simulink model "Commande_3_Changement_de_base_et_diffeomorphisme_"  (R2015a)
settings: Solver=ode45  StartTime=0.0  StopTime=15  MaxStep=0.001  RelTol=1e-3
values from neighbouring files (symbols this model uses):
  Ks = K(:,4)    [A_2_Changement_de_base_Diphiomorphisme.m]
  Kw = K( : , 1:3 )    [A_2_Changement_de_base_Diphiomorphisme.m]
undefined symbols (not defined in the file or in its folder): sfun3d
settings Model: Creator=user  LastModifiedBy=user

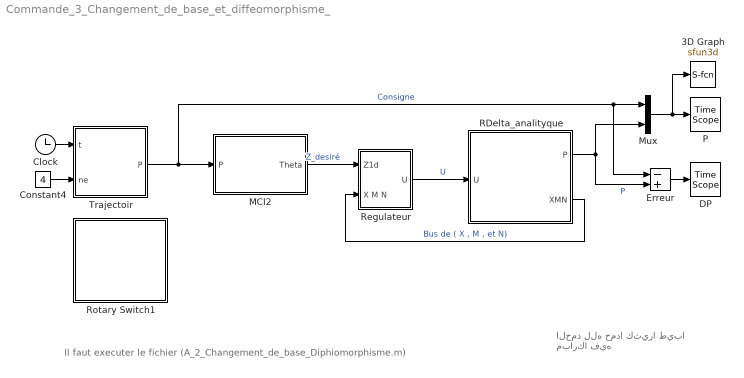
== system Commande_3_Changement_de_base_et_diffeomorphisme_ ==
  note: Il faut executer le fichier (A_2_Changement_de_base_Diphiomorphisme.m)
  note: الحمد لله حمدا كثيرا طيبا مباركا فيه
  3D Graph : S-Function  LoadFcn=sfun3d([],[],[],'LoadBlock')  StartFcn=sfun3d([],[],[],'Start')  StopFcn=sfun3d([],[],[],'Stop')  FunctionName=sfun3d  Parameters=ax,T,np,cp,gd,ls,mk  mask(3D Graph){np=2, ax=[-1 1 -1 1 -2 0]*0.3, cp=[3 2 1], gd=on, ls=-, mk=none, T=0.0001}
      mask prompts: np "Number of point (lines)"; ax "[xmin xmax  ymin ymax zmin zmax]"; cp "Camera position (use [0 0 1] for 2D XY view)"; gd "Grid (on|off)"; ls "LineStyle"; mk "Marker"; T "Sampling Time"
      mask help:
      | This block plots the position of several points in the XYZ space. The input contains the coordinates of all the points (x1,y1,z1,x2,y2,z2,...).
      | The number of points (lines), the XYZ ranges, camera position, grid, linestyle, marker and sampling time, can be set as mask parameters.
      settings: CopyFcn=sfun3d([],[],[],'CopyBlock')  DeleteFcn=sfun3d([],[],[],'DeleteBlock')  NameChangeFcn=sfun3d([],[],[],'NameChange')
      mask Help:
      | This block plots the position of several points in the XYZ space. The input contains the coordinates of all the points (x1,y1,z1,x2,y2,z2,...).
      | The number of points (lines), the XYZ ranges, camera position, grid, linestyle, marker and sampling time, can be set as mask parameters.
      mask TypeOptions ls: - | -- | : | -. | none
      mask TypeOptions mk: none | . | + | o | * | x | square | diamond | v | ^ | > | < | pentagram | hexagram
      mask Display: plot([.05 .95 .95 .05 .05],[.45 .45 .95 .95 .45], 0.5+cos(0:0.1:2*pi)*0.3,0.7+sin(0:0.1:2*pi)*0.2)
  Clock : Clock
  Constant4 : Constant  Value=4
  DP : TimeScope  DefaultConfigurationName=spbscopes.TimeScopeBlockCfg
  Erreur : Sum  Inputs=-+
  MCI2 : MATLAB Function  TreatAsAtomicUnit=on
  Mux : Mux  Inputs=2
  P : TimeScope  DefaultConfigurationName=spbscopes.TimeScopeBlockCfg
  RDelta_analityque : Subsystem
      mask Display:
      | image(imread('DeltaImage2.PNG'))
      | 
      | port_label('input',1,'U')
      | 
      | port_label('output',1,'P')
      | 
      | port_label('output',2,'XMN')
  Regulateur : Subsystem
  Rotary Switch1 : Subsystem  DialogController=hmiCreateDDGDialog  IsWebBlock=on  mask(MathWorksWebBlock){webBlockId=e030fcf6-dd97-4258-a719-13022b0e8ecf, webBlockType=discreteknob, ShowInLibBrowser=on, ShowInitialText=on, HMISrcModelName=Commande_3_Changement_de_base_et_diffeomorphisme_}
      mask prompts: webBlockId "WebBlock Id"; webBlockType "WebBlock Type"; HMISrcModelName "Source Model"
      mask Help: helpview([docroot '/mapfiles/simulink.map'], 'hmi_rotary_switch')
      mask Display:
      | model = bdroot(gcb);
      | if strcmp(get_param(model,'BlockDiagramType'), 'library')
      |     image([(matlabroot) '/toolbox/simulink/hmi/icons/DiscreteKnob.png']);
      | end
  Trajectoir : MATLAB Function  TreatAsAtomicUnit=on
  wires:
  RDelta_analityque/1(P) -> Erreur/2, Mux/2  "P"
  Mux/1 -> P/1, 3D Graph/1
  RDelta_analityque/2(XMN) -> Regulateur/2(X M N)  "Bus de ( X , M , et N)"
  Regulateur/1(U) -> RDelta_analityque/1(U)  "U"
  Trajectoir/1(P) -> MCI2/1(P), Mux/1, Erreur/1  "Consigne"
  Clock/1 -> Trajectoir/1(t)
  Constant4/1 -> Trajectoir/2(ne)
  MCI2/1(Theta) -> Regulateur/1(Z1d)  "Z_desiré"
  Erreur/1 -> DP/1

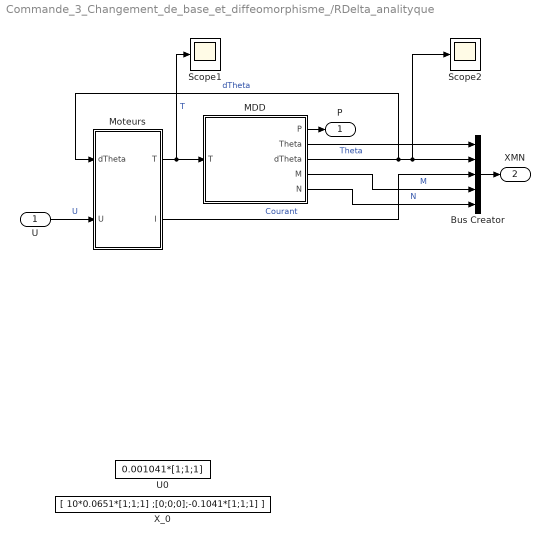
== system Commande_3_Changement_de_base_et_diffeomorphisme_/RDelta_analityque ==
  U : Inport
  Bus Creator : BusCreator  Inputs=5
  MDD : Subsystem
      mask Display:
      | image(imread('DeltaImage2.PNG'))
      | port_label('input',1,'T')
      | port_label('output',1,'P')
      | port_label('output',2,'Theta')
      | port_label('output',3,'dTheta')
      | port_label('output',4,'M')
      | port_label('output',5,'N')
  Moteurs : Subsystem
      mask Display:
      | image('image_motor.jpg')
      | port_label('output',1,'T')
      | port_label('output',2,'I')
      | port_label('input',1,'U')
      | port_label('input',2,'dTheta')
  Scope1 : Scope
      settings: YMin=-0.2  YMax=0.175  SaveName=ScopeData3
  Scope2 : Scope
      settings: YMin=0.774525  YMax=0.774531  SaveName=ScopeData7
  U0 : Constant  Value=0.001041*[1;1;1]
  X_0 : Constant  Value=[ 10*0.0651*[1;1;1] ;[0;0;0];-0.1041*[1;1;1] ]
  P : Outport
  XMN : Outport  Port=2
  wires:
  Moteurs/2(I) -> Bus Creator/3  "Courant"
  U/1 -> Moteurs/2(U)  "U"
  MDD/2(Theta) -> Bus Creator/1  "Theta"
  MDD/3(dTheta) -> Moteurs/1(dTheta), Bus Creator/2, Scope2/1  "dTheta"
  Moteurs/1(T) -> Scope1/1, MDD/1(T)  "T"
  MDD/1(P) -> P/1
  MDD/4(M) -> Bus Creator/4  "M"
  MDD/5(N) -> Bus Creator/5  "N"
  Bus Creator/1 -> XMN/1

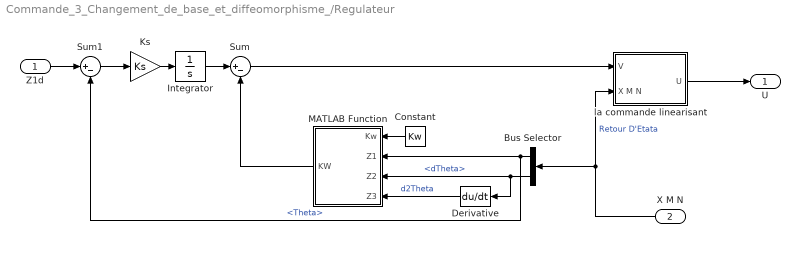
== system Commande_3_Changement_de_base_et_diffeomorphisme_/Regulateur ==
  Z1d : Inport
  X M N : Inport  Port=2
  Bus Selector : BusSelector  OutputSignals=Theta,dTheta
  Constant : Constant  Value=Kw
  Derivative : Derivative
  Integrator : Integrator
  Ks : Gain  Gain=Ks
  MATLAB Function : MATLAB Function  TreatAsAtomicUnit=on
  Sum : Sum  Inputs=|+-
  Sum1 : Sum  Inputs=|+-
  la commande linearisant : Subsystem
  U : Outport
  wires:
  la commande linearisant/1(U) -> U/1
  Derivative/1 -> MATLAB Function/4(Z3)  "d2Theta"
  Bus Selector/1 -> MATLAB Function/2(Z1), Sum1/2  "<Theta>"
  X M N/1 -> Bus Selector/1, la commande linearisant/2(X M N)  "Retour D'Etata"
  Bus Selector/2 -> MATLAB Function/3(Z2), Derivative/1  "<dTheta>"
  Ks/1 -> Integrator/1
  MATLAB Function/1(KW) -> Sum/2
  Sum/1 -> la commande linearisant/1(V)
  Integrator/1 -> Sum/1
  Z1d/1 -> Sum1/1
  Sum1/1 -> Ks/1
  Constant/1 -> MATLAB Function/1(Kw)

== system Commande_3_Changement_de_base_et_diffeomorphisme_/Rotary Switch1 ==

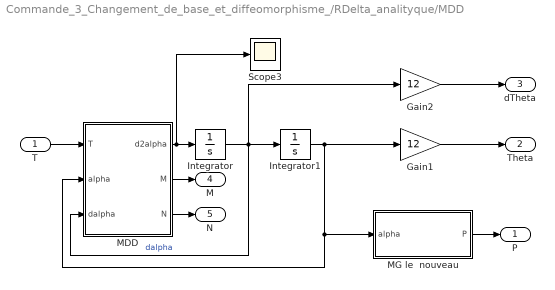
== system Commande_3_Changement_de_base_et_diffeomorphisme_/RDelta_analityque/MDD ==
  T : Inport
  Gain1 : Gain  Gain=12
  Gain2 : Gain  Gain=12
  Integrator : Integrator  InitialCondition=[0;0;0]
  Integrator1 : Integrator  InitialCondition=0.8*[1;1;1]/12
  MDD : Subsystem
  MG le  nouveau : MATLAB Function  TreatAsAtomicUnit=on
  Scope3 : Scope
      settings: TimeRange=2.077341948455237  YMin=0.00075  YMax=0.00275  SaveName=ScopeData2
  P : Outport
  Theta : Outport  Port=2
  dTheta : Outport  Port=3
  M : Outport  Port=4
  N : Outport  Port=5
  wires:
  MDD/1(d2alpha) -> Scope3/1, Integrator/1
  Integrator/1 -> Gain2/1, MDD/3(dalpha), Integrator1/1  "dalpha"
  Integrator1/1 -> MG le  nouveau/1(alpha), MDD/2(alpha), Gain1/1
  T/1 -> MDD/1(T)
  MG le  nouveau/1(P) -> P/1
  Gain1/1 -> Theta/1
  Gain2/1 -> dTheta/1
  MDD/2(M) -> M/1
  MDD/3(N) -> N/1

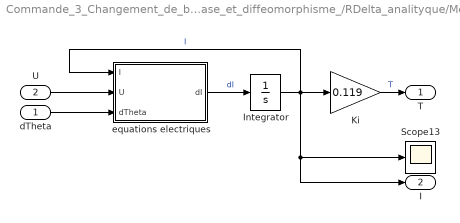
== system Commande_3_Changement_de_base_et_diffeomorphisme_/RDelta_analityque/Moteurs ==
  dTheta : Inport
  U : Inport  Port=2
  Integrator : Integrator  InitialCondition=0*[1;1;1]
  Ki : Gain  Gain=0.119
  Scope13 : Scope
      settings: TimeRange=0.507510643892459  YMin=-1000  YMax=1000  SaveName=ScopeData24
  equations electriques : MATLAB Function  TreatAsAtomicUnit=on
  T : Outport
  I : Outport  Port=2
  wires:
  U/1 -> equations electriques/2(U)
  Integrator/1 -> Scope13/1, I/1, Ki/1, equations electriques/1(I)  "I"
  equations electriques/1(dI) -> Integrator/1  "dI"
  dTheta/1 -> equations electriques/3(dTheta)
  Ki/1 -> T/1  "T"

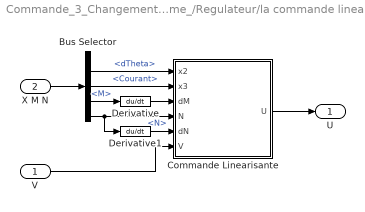
== system Commande_3_Changement_de_base_et_diffeomorphisme_/Regulateur/la commande linearisant ==
  V : Inport
  X M N : Inport  Port=2
  Bus Selector : BusSelector  OutputSignals=Theta,dTheta,Courant,M,N
  Commande Linearisante : MATLAB Function  TreatAsAtomicUnit=on
  Derivative : Derivative
  Derivative1 : Derivative
  U : Outport
  wires:
  X M N/1 -> Bus Selector/1
  Bus Selector/2 -> Commande Linearisante/1(x2)  "<dTheta>"
  Bus Selector/3 -> Commande Linearisante/2(x3)  "<Courant>"
  Derivative/1 -> Commande Linearisante/3(dM)
  Bus Selector/4 -> Derivative/1  "<M>"
  Derivative1/1 -> Commande Linearisante/5(dN)
  Bus Selector/5 -> Derivative1/1, Commande Linearisante/4(N)  "<N>"
  V/1 -> Commande Linearisante/6(V)
  Commande Linearisante/1(U) -> U/1

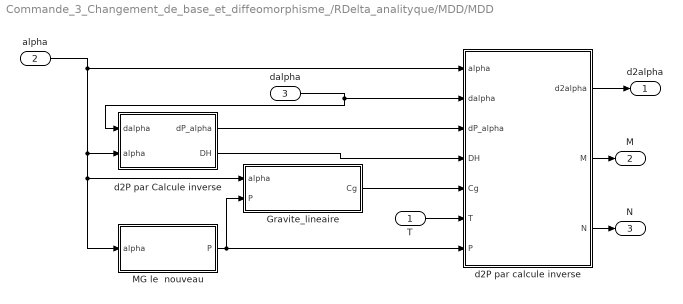
== system Commande_3_Changement_de_base_et_diffeomorphisme_/RDelta_analityque/MDD/MDD ==
  T : Inport
  alpha : Inport  Port=2
  dalpha : Inport  Port=3
  Gravite_lineaire : MATLAB Function  TreatAsAtomicUnit=on
  MG le  nouveau : MATLAB Function  TreatAsAtomicUnit=on
  "d2P par Calcule inverse " : Subsystem
  d2P par calcule inverse : MATLAB Function  TreatAsAtomicUnit=on
  d2alpha : Outport
  M : Outport  Port=2
  N : Outport  Port=3
  wires:
  d2P par calcule inverse/1(d2alpha) -> d2alpha/1
  "d2P par Calcule inverse "/1(dP_alpha) -> d2P par calcule inverse/3(dP_alpha)
  "d2P par Calcule inverse "/2(DH) -> d2P par calcule inverse/4(DH)
  MG le  nouveau/1(P) -> Gravite_lineaire/2(P), d2P par calcule inverse/7(P)
  dalpha/1 -> "d2P par Calcule inverse "/1(dalpha), d2P par calcule inverse/2(dalpha)
  alpha/1 -> MG le  nouveau/1(alpha), Gravite_lineaire/1(alpha), "d2P par Calcule inverse "/2(alpha), d2P par calcule inverse/1(alpha)
  Gravite_lineaire/1(Cg) -> d2P par calcule inverse/5(Cg)
  T/1 -> d2P par calcule inverse/6(T)
  d2P par calcule inverse/2(M) -> M/1
  d2P par calcule inverse/3(N) -> N/1

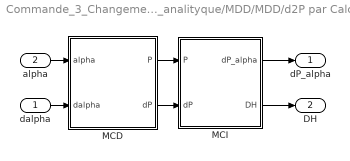
== system Commande_3_Changement_de_base_et_diffeomorphisme_/RDelta_analityque/MDD/MDD/d2P par Calcule inverse  ==
  dalpha : Inport
  alpha : Inport  Port=2
  MCD : MATLAB Function  TreatAsAtomicUnit=on
  MCI : MATLAB Function  TreatAsAtomicUnit=on
  dP_alpha : Outport
  DH : Outport  Port=2
  wires:
  MCD/2(dP) -> MCI/2(dP)
  MCD/1(P) -> MCI/1(P)
  alpha/1 -> MCD/1(alpha)
  dalpha/1 -> MCD/2(dalpha)
  MCI/1(dP_alpha) -> dP_alpha/1
  MCI/2(DH) -> DH/1

== matlab function Commande_3_Changement_de_base_et_diffeomorphisme_/RDelta_analityque/MDD/MDD/MG le  nouveau ==
  data: alpha input; P output
function P =MGD(alpha)


alpha1=alpha(1) ;alpha2=alpha(2) ; alpha3=alpha(3) ;

%les constantes
l1 = 0.19992; 
l2 = 0.334; 
r = 0.126; 
phi2 = 2*pi/3;
phi3 = 4*pi/3;

%% Les points :
C1=[r+l1*cos(alpha1) ; 0 ; -l1*sin(alpha1) ]; 
C2=[(r+l1*cos(alpha2))*cos(phi2) ; (r+l1*cos(alpha2))*sin(phi2) ; -l1*sin(alpha2) ]; 
C3=[(r+l1*cos(alpha3))*cos(phi3) ; (r+l1*cos(alpha3))*sin(phi3) ; -l1*sin(alpha3) ]; 

%% Les vecteurs du triangle C1C2C3 et ses distances
C1C2= C2-C1 ; C2C3 =C3-C2 ; C3C1= C1-C3 ;
a=sqrt(C1C2'*C1C2) ; b=sqrt(C2C3'*C2C3)  ; c=sqrt(C3C1'*C3C1)  ;
 p= a+b+c ; % Le perimetre de C1C2C3
 R = a*b*c/sqrt(p*(p-2*a)*(p-2*b)*(p-2*c)) ;

 %% Calcule du point L 
 % Les vecteurs u et n:
 v1=C1C2/a ;
 n=cross(C3C1,C1C2)*2*R/(a*b*c) ;
 TL = sqrt(R^2-a^2/4) ;
 OL=(C1+C2)/2+TL*sign(-a*a+c*c+b*b)*cross(n,v1);
 %% Calcule du point E :
P=OL-sqrt(l2^2-R^2)*n ;

== matlab function Commande_3_Changement_de_base_et_diffeomorphisme_/MCI2 ==
  data: P input; Theta output
    function Theta = fcn(P)

    l1 = 0.19992; 
    l2 = 0.334; 
    r = 0.126; 
    phi2 = 2*pi/3;
    phi3 = 4*pi/3;

    %% Expression de P dans Ri
    % l'expression P1 dP1 et d2P1 ne se changent pas
    A2=[cos(phi2) sin(phi2) 0
        -sin(phi2) cos(phi2) 0
        0            0      1 ]; 
    A3=[cos(phi3) sin(phi3) 0
        -sin(phi3) cos(phi3) 0
        0            0      1 ];
     P2=A2*P; 
     P3=A3*P ; 
        
    x1=P(1); y1=P(2) ; z1=P(3) ; 
    x2=P2(1); y2=P2(2) ; z2=P2(3) ;
    x3=P3(1); y3=P3(2) ; z3=P3(3) ;
   
    % L'expression de dP dans Ri :
      

    %% Parametres du Triangle AiCiBi :
    % Triangle 1 :
    AB1=sqrt(z1^2+(x1-r)^2);
    e1=sqrt(l2^2-y1^2); 
    AB2=sqrt(z2^2+(x2-r)^2);
    e2=sqrt(l2^2-y2^2);
    AB3=sqrt(z3^2+(x3-r)^2);
    e3=sqrt(l2^2-y3^2);

    %% calcul de alpha1
    beta1=atan2(-z1,x1-r);
    delta1=acos((AB1^2 + l1^2 - e1^2)/(2*l1*AB1));
    alpha1=beta1-delta1; 


    %% calcul de alpha2
    beta2=atan2(-z2,x2-r);
    delta2=acos((AB2^2 + l1^2 - e2^2)/(2*l1*AB2));
    alpha2=beta2-delta2; 


    %% calcul de alpha3
    beta3=atan2(-z3,x3-r);
    delta3=acos((AB3^2 + l1^2 - e3^2)/(2*l1*AB3));
    alpha3=beta3-delta3; 

% Tranformation au Deg
alpha=[alpha1;alpha2;alpha3]; % first solution
Theta=12*alpha;

== matlab function Commande_3_Changement_de_base_et_diffeomorphisme_/RDelta_analityque/MDD/MDD/d2P par Calcule inverse /MCD ==
  data: P output; alpha input; dalpha input; dP output
function [P,dP]= fcn(alpha,dalpha)

% alpha=alpha*pi/180;
% dalpha=dalpha*pi/180;
% d2alpha=d2alpha*pi/180;
alpha1=alpha(1) ;alpha2=alpha(2) ; alpha3=alpha(3) ;
dalpha1=dalpha(1) ;dalpha2=dalpha(2) ; dalpha3=dalpha(3) ;

%% Remarque: une letrre majiscule signifie un point ou un vecteur 
% tandit que un miniscule signifie la norme
%% les constantes
l1 = 0.19992; 
l2 = 0.334; 
r = 0.126; 
phi2 = 2*pi/3;
phi3 = 4*pi/3;
% Fin
%% les points Ci :
OC1=[r+l1*cos(alpha1) ; 0 ; -l1*sin(alpha1) ]; 
OC2=[(r+l1*cos(alpha2))*cos(phi2) ; (r+l1*cos(alpha2))*sin(phi2) ; -l1*sin(alpha2) ]; 
OC3=[(r+l1*cos(alpha3))*cos(phi3) ; (r+l1*cos(alpha3))*sin(phi3) ; -l1*sin(alpha3) ]; 
%% Les veccteurs CiCj :
C1C2=OC2-OC1; C2C3=OC3-OC2 ; C3C1=OC1-OC3;
%% vitesses de point Ci et CiCj:
% dC1= Q1*dAlpha1;
Q1=[-l1*sin(alpha1) ; 0 ; -l1*cos(alpha1)] ; 
Q2=[-l1*sin(alpha2)*cos(phi2) ; -l1*sin(alpha2)*sin(phi2) ; -l1*cos(alpha2)] ;
Q3=[-l1*sin(alpha3)*cos(phi3) ; -l1*sin(alpha3)*sin(phi3) ; -l1*cos(alpha3)] ;
dOC1=Q1*dalpha1 ;
dOC2=Q2*dalpha2 ;
dOC3=Q3*dalpha3 ;
dC1C2=dOC2-dOC1 ; dC2C3=dOC3-dOC2 ; dC3C1=dOC1-dOC3 ;

%% Les longueurs a,b,et c:
a=sqrt(C1C2'*C1C2);
b=sqrt(C2C3'*C2C3);
c=sqrt(C3C1'*C3C1);

%% Calcule de R et s :
p=a+b+c ; % le perimetre
p1=p-2*a ; p2=p-2*b ;  p3=p-2*c ; 
R=a*b*c/sqrt(p*p1*p2*p3); % le Rayon du C1C2C3
s=a*b*c/(2*R); % La surface
V1=C1C2/a; % les vecteures unitaires portes sur les segments
V2=C2C3/b;
V3=C3C1/c;
%% Calcule de n et w:
n=cross(C3C1,C1C2)/s ; % le Vecteur normale
w=sign(-a*a+c*c+b*b)*cross(n,V1) ;
%% les segments  tl=|TK| , ml=|ML| ,lp=|LP|
tl=sqrt(R^2-(a/2)^2);
ml=sqrt(R^2-(b/2)^2);
kl=sqrt(R^2-(c/2)^2);
lp=sqrt(l2^2-R^2) ;
%% les vitess de a,b,et c:
da=V1'*dC1C2;
db=V2'*dC2C3;
dc=V3'*dC3C1;
%% Calcule de dR:
dp=da+db+dc ;
dp1=dp-2*da ; dp2=dp-2*db ; dp3=dp-2*dc ;
dR = ( da/a + db/b + dc/c - 0.5*( dp/p + dp1/p1 + dp2/p2 + dp3/p3 ))*R ;
%dR = ( 1 - 4*R*tl/b/c)*R*da/a + (1-4*R*ml/a/c)*R*db/b + (1-4*R*kl/a/b)*R*dc/c ;
%% Calcule de :
dtl=(R*dR-a*da/4)/tl ;
dlp  = -R*dR/lp ;
ds = (da/a + db/b + dc/c - dR/R)*s ;
dV1=(dC1C2-da*V1)/a ;

dS = cross(dC3C1,C1C2) + cross(C3C1,dC1C2) ;
dn= (dS-ds*n)/s ;
dw=sign(-a*a+c*c+b*b)*(cross(dn,V1) + cross(n,dV1)) ;
% Calcule de P :
OL = (OC1+OC2)/2 + tl*w;
P = OL-lp*n ;
% Calcule de dP :
dOT = (dOC2 + dOC1)/2 ; 
dTL = dtl*w + tl*dw ;
dLP = -dlp*n - lp*dn ; 
dP = dOT + dTL + dLP ;

== matlab function Commande_3_Changement_de_base_et_diffeomorphisme_/Regulateur/la commande linearisant/Commande Linearisante ==
  data: x2 input; x3 input; dM input; N input; U output; dN input; V input
function U = fcn(x2,x3,dM,N,dN,V)

%% Mode glissant
% Les Constantes des moteurs ;
b1 = -1.1250e+03 ;
b2 = -99.4718 ;
b3 =833.3333 ;
%Constantes du Reglage :

U=(N\(-dM-dN*x3+V)-b2*x2-b1*x3)/b3 ;

== matlab function Commande_3_Changement_de_base_et_diffeomorphisme_/Regulateur/MATLAB Function ==
  data: Kw input; Z1 input; KW output; Z2 input; Z3 input
function KW = RE(Kw,Z1,Z2,Z3)

% Les sous systemes correspendants aux moteurs 1,2 et 3
w1 = [Z1(1);Z2(1);Z3(1)] ; 
w2 = [Z1(2);Z2(2);Z3(2)] ;
w3 = [Z1(3);Z2(3);Z3(3)] ;
% Les retour d'etat
KW1 = Kw'*w1 ; KW2 = Kw'*w2 ; KW3 = Kw'*w3 ;
KW= [KW1 ; KW2 ; KW3 ] ;

== matlab function Commande_3_Changement_de_base_et_diffeomorphisme_/RDelta_analityque/MDD/MDD/Gravite_lineaire ==
  data: alpha input; Cg output; P input
function Cg = fcn(alpha,P)

    alpha1=alpha(1) ;alpha2=alpha(2) ; alpha3=alpha(3) ;
    
%% les constantes:
l1 = 0.19992; 
l2 = 0.334; 
r = 0.126; 
phi2 = 2*pi/3;
phi3 = 4*pi/3;
A2=[cos(phi2) sin(phi2) 0 
     -sin(phi2) cos(phi2) 0
        0            0            1 ]; 
A3=[cos(phi3) sin(phi3) 0
     -sin(phi3) cos(phi3) 0
          0            0          1 ];
g = 9.98 ;
mBras = 0.083660682814532691 ;
mRoue =0.1805;
dBras = 0.058869490365843639 ;
dRoue = 0.0344586;
M2= 2*0.01438 ;
M3 = 0.0416;
shift = 0.0651;
%% Parametres :
    % A) les vecteurs OAi et OBi :
    OA1=[r ; 0 ; 0] ; OA2=[r*cos(phi2) ; r*sin(phi2) ; 0] ; OA3=[r*cos(phi3) ; r*sin(phi3) ; 0] ;
    OC1=[r+l1*cos(alpha1) ; 0 ; -l1*sin(alpha1) ]; 
    OC2=[(r+l1*cos(alpha2))*cos(phi2) ; (r+l1*cos(alpha2))*sin(phi2) ; -l1*sin(alpha2) ]; 
    OC3=[(r+l1*cos(alpha3))*cos(phi3) ; (r+l1*cos(alpha3))*sin(phi3) ; -l1*sin(alpha3) ]; 
    % B) Les vecteurs AiCi :
    A1C1=OC1-OA1 ; A2C2=OC2-OA2 ; A3C3=OC3-OA3 ;
    % Fin

%% ===============-------=====  Calcule de Cgi =====---------====================

% Les vecteurs unitaires portes par les bras paralleles : la nouvelle base
    u1=(P-OC1)/l2 ; u2=(P-OC2)/l2 ; u3=(P-OC3)/l2 ;
    U = [u1 u2 u3] ;

% Les forces aux points Ci ;
     N1=[-dBras*mBras*sin(shift) - dRoue*mRoue*cos(shift) ; 0 ; -dBras*mBras*cos(shift) + dRoue*mRoue*sin(shift)]*g/l1; 
    N2=[0 ;0 ; -M2*g/2] ;
    N=N1+N2;

% les effets totales appliquees a  la nacelle (N4):
    N4 = [0 ; 0 ; -(M3 + M2*3/2)*g] ;

% les composants de N4 sur les bras paralleles = Expression de N4 dans la Nouvelle base U:
    E1 = [1 0 0]; E2 = [0 1 0]; E3 = [0 0 1];
    Z = U\N4 ;
    Z1=(E1*Z)*u1; 
    Z2=(E2*Z)*u2;  
    Z3=(E3*Z)*u3 ;

% les matrices de transformation au plan OXiZi (Bi) :
    B1= [1 0 0; 0 0 0 ; 0 0 1] ;
    B2=B1*A2; B3=B1*A3 ;
% Le couple Cg1 au point de fonc P0:
Cg1 = E2*cross(A1C1,N + B1*Z1);
Cg2 = E2* cross(A2*A2C2,N + B2*Z2)  ;
Cg3 = E2* cross(A3*A3C3, N + B3*Z3) ;
Cg =[Cg1 ;Cg2;Cg3] ;

== matlab function Commande_3_Changement_de_base_et_diffeomorphisme_/RDelta_analityque/MDD/MDD/d2P par Calcule inverse /MCI ==
  data: P input; dP input; dP_alpha output; DH output
    function [dP_alpha,DH]= fcn(P,dP)

    l1 = 0.19992; 
    l2 = 0.334; 
    r = 0.126; 
    phi2 = 2*pi/3;
    phi3 = 4*pi/3;

    %% Expression de P dans Ri
    % l'expression P1 dP1 et d2P1 ne se changent pas
    A2=[cos(phi2) sin(phi2) 0
        -sin(phi2) cos(phi2) 0
        0            0      1 ]; 
    A3=[cos(phi3) sin(phi3) 0
        -sin(phi3) cos(phi3) 0
        0            0      1 ];
     P2=A2*P; dP2=A2*dP; 
     P3=A3*P ; dP3=A3*dP ; 
        
    x1=P(1); y1=P(2) ; z1=P(3) ; 
    x2=P2(1); y2=P2(2) ; z2=P2(3) ;
    x3=P3(1); y3=P3(2) ; z3=P3(3) ;
   
    %% Parametres du Triangle AiCiBi :
    % Triangle 1 :
    AB1=sqrt(z1^2+(x1-r)^2);
    e1=sqrt(l2^2-y1^2); 
    AB2=sqrt(z2^2+(x2-r)^2);
    e2=sqrt(l2^2-y2^2);
    AB3=sqrt(z3^2+(x3-r)^2);
    e3=sqrt(l2^2-y3^2);

    %% calcul de alpha1
    beta1=atan2(-z1,x1-r);
    delta1=acos((AB1^2 + l1^2 - e1^2)/(2*l1*AB1));
    alpha1=beta1-delta1; 


    %% calcul de alpha2
    beta2=atan2(-z2,x2-r);
    delta2=acos((AB2^2 + l1^2 - e2^2)/(2*l1*AB2));
    alpha2=beta2-delta2; 


    %% calcul de alpha3
    beta3=atan2(-z3,x3-r);
    delta3=acos((AB3^2 + l1^2 - e3^2)/(2*l1*AB3));
    alpha3=beta3-delta3; 

% Tranformation au Deg
alpha=[alpha1;alpha2;alpha3]; % first solution


%% =================== Calcule de dalpha_i ====================================

% ---------------------------- Calcul de dAlpha1 ----------------------
% Calcule de dDelta1 :
BH1 = AB1-l1*cos(delta1);
D1=l1*AB1*sin(delta1) ;
dDelta1X = -BH1*(x1-r)/AB1/D1 ; 
dDelta1Y = -y1/D1 ; 
dDelta1Z = -BH1*z1/AB1/D1 ; 
Gdelta1=  [ dDelta1X , dDelta1Y , dDelta1Z] ;
dDelta1 = Gdelta1*dP ;
% Calcule de dBeta1 :
dBeta1Z=-(x1-r)/AB1^2 ; dBeta1X=z1/AB1^2 ;
Gbeta1=[ dBeta1X ,  0 , dBeta1Z] ;
dBeta1 = Gbeta1*dP;
% Calcule de dAlpha1 :
Galpha1=Gbeta1-Gdelta1 ;
dAlpha1 = Galpha1*dP ;

% ---------------------------- Calcul de dAlpha2 ----------------------
% Calcule de dDelta2 :
BH2 = AB2-l1*cos(delta2);
D2=l1*AB2*sin(delta2) ;
dDelta2X = -BH2*(x2-r)/AB2/D2 ; 
dDelta2Y = -y2/D2 ; 
dDelta2Z = -BH2*z2/AB2/D2 ; 
Gdelta2=  [ dDelta2X , dDelta2Y , dDelta2Z] ;
dDelta2 = Gdelta2*dP2 ;
% Calcule de dBeta2 :
dBeta2Z=-(x2-r)/AB2^2 ; dBeta2X=z2/AB2^2 ;
Gbeta2=[ dBeta2X ,  0 , dBeta2Z] ;
dBeta2 = Gbeta2*dP2;
% Calcule de dAlpha2 :
Galpha2=Gbeta2-Gdelta2 ;
dAlpha2 = Galpha2*dP2 ;

% ---------------------------- Calcul de dAlpha3 ----------------------
% Calcule de dDelta2 :
BH3 = AB3-l1*cos(delta3);
D3=l1*AB3*sin(delta3) ;
dDelta3X = -BH3*(x3-r)/AB3/D3 ; 
dDelta3Y = -y3/D3 ; 
dDelta3Z = -BH3*z3/AB3/D3 ; 
Gdelta3=  [ dDelta3X , dDelta3Y , dDelta3Z] ;
dDelta3 = Gdelta3*dP3 ;
% Calcule de dBeta3:
dBeta3Z=-(x3-r)/AB3^2 ; dBeta2X=z3/AB3^2 ;
Gbeta3=[ dBeta2X ,  0 , dBeta3Z] ;
dBeta3 = Gbeta3*dP3;
% Calcule de dAlpha3 :
Galpha3=Gbeta3-Gdelta3 ;
dAlpha3 = Galpha3*dP3 ;

dalpha=[ dAlpha1 ; dAlpha2 ; dAlpha3 ];

%% ===================== Calcule de d2alpha_i =================================
 
% ---------------------------- Calcul de d2Alpha1 ----------------------
% Calcule de d2Gama1 :
CH1=l1*sin(delta1);
AH1=l1*cos(delta1) ;
d2Delta1XX = -BH1*(x1-r)^2/(AB1^3*D1)*( AH1*e1^2/(BH1*CH1^2) + (AB1/(x1-r))^2 - 2 ) ;
d2Delta1YY = - (1+y1^2*AH1*AB1/D1^2 )  /D1;
d2Delta1ZZ  = -BH1*z1^2/(AB1^3*D1)*( AH1*e1^2/(BH1*CH1^2) + (AB1/z1)^2 -2 ) ;
d2Delta1XY = y1*(x1-r)*(CH1^2-AH1*BH1)/D1^3 ;
d2Delta1XZ = -BH1*(x1-r)*z1/(AB1^3*D1)*( AH1*e1^2/(BH1*CH1^2) - 2 ) ;
d2Delta1YZ = y1*z1*(CH1^2-AH1*BH1)/D1^3 ; 
Hdelta1=[ d2Delta1XX,d2Delta1XY,d2Delta1XZ ; d2Delta1XY, d2Delta1YY,d2Delta1YZ ;d2Delta1XZ , d2Delta1YZ,d2Delta1ZZ] ;

%Calcule de dBeta 1:
d2Beta1XX=-2*(x1-r)*z1/AB1^4 ; d2Beta1ZZ=-d2Beta1XX ; d2Beta1XZ = ((x1-r)^2-z1^2)/AB1^4 ;
Hbeta1= [d2Beta1XX , 0, d2Beta1XZ ; 0, 0, 0 ; d2Beta1XZ , 0 , d2Beta1ZZ ] ;

%Calcule de dAlpha1 :
Halpha1= Hbeta1 - Hdelta1; 


% ---------------------------- Calcul de d2Alpha2 ----------------------
% Calcule de d2Gama1 :
CH2=l1*sin(delta2);
AH2=l1*cos(delta2) ;
d2Delta2XX = -BH2*(x2-r)^2/(AB2^3*D2)*( AH2*e2^2/(BH2*CH2^2) + (AB2/(x2-r))^2 - 2 ) ;
d2Delta2YY = - (1+y2^2*AH2*AB2/D2^2 )  /D2;
d2Delta2ZZ  = -BH2*z2^2/(AB2^3*D2)*( AH2*e2^2/(BH2*CH2^2) + (AB2/z2)^2 -2 ) ;
d2Delta2XY = y2*(x2-r)*(CH2^2-AH2*BH2)/D2^3 ;
d2Delta2XZ = -BH2*(x2-r)*z2/(AB2^3*D2)*( AH2*e2^2/(BH2*CH2^2) - 2 ) ;
d2Delta2YZ = y2*z2*(CH2^2-AH2*BH2)/D2^3 ; 
Hdelta2=[ d2Delta2XX,d2Delta2XY,d2Delta2XZ ; d2Delta2XY, d2Delta2YY,d2Delta2YZ ;d2Delta2XZ , d2Delta2YZ,d2Delta2ZZ] ;

%Calcule de dBeta2:
d2Beta2XX=-2*(x2-r)*z2/AB2^4 ; d2Beta2ZZ=-d2Beta2XX ; d2Beta2XZ = ((x2-r)^2-z2^2)/AB2^4 ;
Hbeta2= [d2Beta2XX , 0, d2Beta2XZ ; 0, 0, 0 ; d2Beta2XZ , 0 , d2Beta2ZZ ] ;

%Calcule de dAlpha2 :
Halpha2= Hbeta2 - Hdelta2; 


% ---------------------------- Calcul de d2Alpha3 ----------------------
% Calcule de d2Gama3 :
CH3=l1*sin(delta3);
AH3=l1*cos(delta3) ;
d2Delta3XX = -BH3*(x3-r)^2/(AB3^3*D3)*( AH3*e3^2/(BH3*CH3^2) + (AB3/(x3-r))^2 - 2 ) ;
d2Delta3YY = - (1+y3^2*AH3*AB3/D3^2 )  /D3;
d2Delta3ZZ  = -BH3*z3^2/(AB3^3*D3)*( AH3*e3^2/(BH3*CH3^2) + (AB3/z3)^2 -2 ) ;
d2Delta3XY = y3*(x3-r)*(CH3^2-AH3*BH3)/D3^3 ;
d2Delta3XZ = -BH3*(x3-r)*z3/(AB3^3*D3)*( AH3*e3^2/(BH3*CH3^2) - 2 ) ;
d2Delta3YZ = y3*z3*(CH3^2-AH3*BH3)/D3^3 ; 
Hdelta3=[ d2Delta3XX,d2Delta3XY,d2Delta3XZ ; d2Delta3XY, d2Delta3YY,d2Delta3YZ ;d2Delta3XZ , d2Delta3YZ,d2Delta3ZZ] ;

%Calcule de dBeta3:
d2Beta3XX=-2*(x3-r)*z3/AB3^4 ; d2Beta3ZZ=-d2Beta3XX ; d2Beta3XZ = ((x3-r)^2-z3^2)/AB3^4 ;
Hbeta3= [d2Beta3XX , 0, d2Beta3XZ ; 0, 0, 0 ; d2Beta3XZ , 0 , d2Beta3ZZ ] ;

%Calcule de dAlpha3 :
Halpha3= Hbeta3 - Hdelta3; 


 % d2alpha=[d2Alpha1 ; d2Alpha2 ; d2Alpha3]; ou bien :

H = [dP'*Halpha1*dP ;dP2'*Halpha2*dP2 ;dP3'*Halpha3*dP3 ] ;
D = [Galpha1;Galpha2*A2;Galpha3*A3] ;
dP_alpha =eye(3)/D ;
DH = D\H ;
%% Clacule inverse de d2P :

% d2P =D\d2alpha-D\H ;

== matlab function Commande_3_Changement_de_base_et_diffeomorphisme_/RDelta_analityque/MDD/MDD/d2P par calcule inverse ==
  data: alpha input; dalpha input; dP_alpha input; DH input; d2alpha output; Cg input; T input; P input; M output; N output
function [d2alpha, M,N]= fcn(alpha,dalpha, dP_alpha,DH,Cg,T,P)

alpha1=alpha(1) ;alpha2=alpha(2) ; alpha3=alpha(3) ;
dalpha1=dalpha(1) ;dalpha2=dalpha(2) ; dalpha3=dalpha(3) ;

%% les constantes
    l1 = 0.19992; 
    l2 = 0.334; 
    r = 0.126; 
    phi2 = 2*pi/3;
    phi3 = 4*pi/3;
A2=[cos(phi2) sin(phi2) 0
    -sin(phi2) cos(phi2) 0
    0            0      1 ]; 
A3=[cos(phi3) sin(phi3) 0
    -sin(phi3) cos(phi3) 0
    0            0      1 ];
% Constantes mecaniques
    J1=0.0071126;
    M2=2*0.01438  ;
    J2 = 2*0.00027499613;
    M3 = 0.04157 ;
    M4=2*J2/l2^2 ;
    
% Fin

% les vecteurs OAi et OCi :
OC1=[r+l1*cos(alpha1) ; 0 ; -l1*sin(alpha1) ]; 
OC2=[(r+l1*cos(alpha2))*cos(phi2) ; (r+l1*cos(alpha2))*sin(phi2) ; -l1*sin(alpha2) ]; 
OC3=[(r+l1*cos(alpha3))*cos(phi3) ; (r+l1*cos(alpha3))*sin(phi3) ; -l1*sin(alpha3) ]; 
%fin

% Les vecteurs unitaires portes par les bras paralleles : la nouvelle base
u1=(P-OC1)/l2 ; u2=(P-OC2)/l2 ; u3=(P-OC3)/l2 ;
%la matrice du transformation = La nouvelle base:
U = [u1 u2 u3] ;
%Uinv=inv(U);

%%  accelerations des points Ci :
% dOCi : la derivee partielle de OCi par rapport au alphai
% d2OCi : la deuxieme derivee partielle de OCi par rapport au alphai

dOC1_1=[-l1*sin(alpha1) ; 0 ; -l1*cos(alpha1)] ; 
dOC2_2=[-l1*sin(alpha2)*cos(phi2) ; -l1*sin(alpha2)*sin(phi2) ; -l1*cos(alpha2)] ;
dOC3_3=[-l1*sin(alpha3)*cos(phi3) ; -l1*sin(alpha3)*sin(phi3) ; -l1*cos(alpha3)] ;

d2OC1_1=[-l1*cos(alpha1) ; 0 ; l1*sin(alpha1)] ;
d2OC2_2=[-l1*cos(alpha2)*cos(phi2) ; -l1*cos(alpha2)*sin(phi2) ; l1*sin(alpha2)] ;
d2OC3_3=[-l1*cos(alpha3)*cos(phi3) ; -l1*cos(alpha3)*sin(phi3) ; l1*sin(alpha3)] ;

%Fin

%% ================ Le couple Cai en point de fonctionnement Couple1==================
% Parametres:
a1 = M2/4-M4/2 ; a2= M2/4 + M4/2; a3=M3 +3*a2 ; 
% la matrice de cross(AiCi,...)=aci  "ACi est exprimee dans le repere Ri"
ac1=[ 0 , l1*sin(alpha1) , 0 ; -l1*sin(alpha1) ,0 , -l1*cos(alpha1) ; 0 , l1*cos(alpha1),0]   ;
ac2=[ 0 , l1*sin(alpha2) , 0 ; -l1*sin(alpha2) ,0 , -l1*cos(alpha2) ; 0 , l1*cos(alpha2),0]   ;
ac3=[ 0 , l1*sin(alpha3) , 0 ; -l1*sin(alpha3) ,0 , -l1*cos(alpha3) ; 0 , l1*cos(alpha3),0]   ;
% Les matrices de projection
E1 = [1 0 0]; E2 = [0 1 0]; E3 = [0 0 1];
B1= [1 0 0; 0 0 0 ; 0 0 1] ; B2=B1*A2; B3=B1*A3 ;
%% 1)  Le couple Ca1 : 
G11=a3*(E2*ac1*B1*u1)*(E1/U) + a1*E2*ac1*B1 ;
G12=a1*(E2*ac1*B1*u1)*(E1/U)  ;
G13=a1*(E2*ac1*B1*u1)*(E1/U) + a2*E2*ac1*B1 ;
%Ca1=(J1+G13*dOC1_1)*d2alpha1+ G11*d2P +(G12*dOC2_2)*d2alpha2 + (G12*dOC3_3)*d2alpha3 +G13*d2OC1_1*dalpha1^2+ (G12*d2OC2_2)*dalpha2^2 + (G12*d2OC3_3)*dalpha3^2;
% Ca1 = J1*d2alpha1 + G11*d2P + G12* (d2OC2 +d2OC3) + G13*d2OC1 ;

%% 2)  Le couple Ca2 : 
G21=a3*(E2*ac2*B2*u2)*(E2/U) + a1*E2*ac2*B2 ;
G22=a1*(E2*ac2*B2*u2)*(E2/U)  ;
G23=a1*(E2*ac2*B2*u2)*(E2/U) + a2*E2*ac2*B2 ;
%Ca2=(J1+G23*dOC2_2)*d2alpha2+ G21*d2P +(G22*dOC1_1)*d2alpha1 + (G22*dOC3_3)*d2alpha3 +G23*d2OC2_2*dalpha2^2+ (G22*d2OC1_1)*dalpha1^2 + (G22*d2OC3_3)*dalpha3^2;
%Ca2 = J1*d2alpha2 + G21*d2P + G22* (d2OC1 +d2OC3) + G23*d2OC2 ;

%% 3)  Le couple Ca3 : 
G31=a3*(E2*ac3*B3*u3)*(E3/U) + a1*E2*ac3*B3 ;
G32=a1*(E2*ac3*B3*u3)*(E3/U)  ;
G33=a1*(E2*ac3*B3*u3)*(E3/U) + a2*E2*ac3*B3 ;
%Ca3=(J1+G33*dOC3_3)*d2alpha3+ G31*d2P +(G32*dOC2_2)*d2alpha2 + (G32*dOC1_1)*d2alpha1 + G33*d2OC3_3*dalpha3^2+ (G32*d2OC2_2)*dalpha2^2 + (G32*d2OC1_1)*dalpha1^2;
% Ca3 = J1*d2alpha3 + G31*d2P + G32* (d2OC2 +d2OC1) + G33*d2OC3 ;
% Fin

 %% ============= Calcule inverse de MDD (d2alpha en fonction de Ca ===========

e11= J1+G13*dOC1_1 ; 
e12 = (G12*dOC2_2) ;
e13 = (G12*dOC3_3) ;
b11 = G13*d2OC1_1 ;
b12 = (G12*d2OC2_2) ;
b13 =(G12*d2OC3_3) ;
% Ca1=e11*d2alpha1+e12*d2alpha2 + e13*d2alpha3 +b11*dalpha1^2+ b12*dalpha2^2 + b13*dalpha3^2 + G11*d2P ;

e21 = (G22*dOC1_1) ;
e22 = (J1+G23*dOC2_2) ;
e23 = (G22*dOC3_3) ;
b21 = (G22*d2OC1_1) ;
b22 = G23*d2OC2_2 ;
b23 = (G22*d2OC3_3) ;
% Ca2 = e22*d2alpha2 + e21*d2alpha1 + e23*d2alpha3 +b22*dalpha2^2 + b21*dalpha1^2 + b23*dalpha3^2 + G21*d2P ;

e31 = (G32*dOC1_1) ;
e32 =(G32*dOC2_2) ;
e33 =(J1+G33*dOC3_3);
b31 = (G32*d2OC1_1) ;
b32 =(G32*d2OC2_2) ;
b33 = G33*d2OC3_3 ;
% Ca3=e33*d2alpha3 +e32*d2alpha2 + e31*d2alpha1 + b33*dalpha3^2+ b32*dalpha2^2 + b31*dalpha1^2 + G31*d2P;

e=[e11 , e12 , e13 ; e21 , e22 , e23 ; e31 , e32 , e33] ;
b=[b11 , b12, b13 ; b21 , b22 , b23 ; b31, b32, b33] ;
G = [G11 ; G21 ; G31]  ;
dalphaCarre=[dalpha1^2 ; dalpha2^2; dalpha3^2] ;
% Ca = e*d2alpha + b*dalphaCarre + G*d2P ;
Ki =0.119 ;
N = 12^2*eye(3,3)/(e+G*dP_alpha)*Ki;
M = (e+G*dP_alpha)\(Cg - b*dalphaCarre + G*DH)*12 ;

%% Calcule de d2alpha :
%Ca=12*T +Cg ;
%d2alpha =(e+G*dP_alpha)\12*T +(e+G*dP_alpha)\(Cg  - b*dalphaCarre + G*DH) ; 
d2Theta = M + N*T/Ki ;
d2alpha = d2Theta /12 ;

== matlab function Commande_3_Changement_de_base_et_diffeomorphisme_/RDelta_analityque/MDD/MG le  nouveau ==
  data: alpha input; P output
function P =MGD(alpha)


alpha1=alpha(1) ;alpha2=alpha(2) ; alpha3=alpha(3) ;

%les constantes
l1 = 0.19992; 
l2 = 0.334; 
r = 0.126; 
phi2 = 2*pi/3;
phi3 = 4*pi/3;

%% Les points :
C1=[r+l1*cos(alpha1) ; 0 ; -l1*sin(alpha1) ]; 
C2=[(r+l1*cos(alpha2))*cos(phi2) ; (r+l1*cos(alpha2))*sin(phi2) ; -l1*sin(alpha2) ]; 
C3=[(r+l1*cos(alpha3))*cos(phi3) ; (r+l1*cos(alpha3))*sin(phi3) ; -l1*sin(alpha3) ]; 

%% Les vecteurs du triangle C1C2C3 et ses distances
C1C2= C2-C1 ; C2C3 =C3-C2 ; C3C1= C1-C3 ;
a=sqrt(C1C2'*C1C2) ; b=sqrt(C2C3'*C2C3)  ; c=sqrt(C3C1'*C3C1)  ;
 p= a+b+c ; % Le perimetre de C1C2C3
 R = a*b*c/sqrt(p*(p-2*a)*(p-2*b)*(p-2*c)) ;

 %% Calcule du point L 
 % Les vecteurs u et n:
 v1=C1C2/a ;
 n=cross(C3C1,C1C2)*2*R/(a*b*c) ;
 TL = sqrt(R^2-a^2/4) ;
 OL=(C1+C2)/2+TL*sign(-a*a+c*c+b*b)*cross(n,v1);
 %% Calcule du point E :
P=OL-sqrt(l2^2-R^2)*n ;

== matlab function Commande_3_Changement_de_base_et_diffeomorphisme_/Trajectoir ==
  data: t input; ne input; P output
function P = fcn(t,ne)

%% Menu
% 1 ==> Ligne horizontal
% 2==>  Ligne suivant l'axe oz
% 3==> Cercle
% 4==> Ligne x=y
 z0=-0.08789 ; zpi=-0.3;
B= (z0+zpi)/2 ; A= (z0-zpi)/2 ; 
f = 1; f2 = 5 ;
R=0.2;
%% vers le Plan Z=-0.3
if (t<pi/f && (ne == 1 || ne == 3 ||  ne == 0 || ne == 4 || ne == 5 ||  ne == 6))
n= 2 ; 
elseif( (ne == 4 || ne == 5 ||  ne == 6)  &&  (t<3*pi/2/f) ) % vers le point (0 , R , -0.3)
n=1 ;
else
n =ne ;
end

%% le trajecoir
switch n
    
    case 0
        
        % La position
        x = R*sin(f*t)  ; y=0 ;
        z=  zpi ;
        P = [ x ; y ; z ];
        % La vitess
        dx = f*R*cos(f*t)  ; dy=0 ;
        dz= 0 ;
        dP = [ dx ; dy ; dz ];
        % L'acceleration :
        d2x = -f^2*R*sin(f*t) ; d2y=0 ;
        d2z =  0;
        d2P = [ d2x ; d2y ; d2z ];
        % L'a _coup :
        d3x = -f^3*R*cos(f*t) ; d3y=0 ;
        d3z =  0;
        d3P = [ d3x ; d3y ; d3z ];
    case 1   
        % La position
        y = R*sin(f*t)  ; x=0 ;
        z= zpi  ;
        P = [ x ; y ; z ];
        % La vitess
        dy = f*R*cos(f*t)  ; dx=0 ;
        dz= 0 ;
        dP = [ dx ; dy ; dz ];
        % L'acceleration :
        d2y = -f^2*R*sin(f*t) ; d2x=0 ;
        d2z =  0;
        d2P = [ d2x ; d2y ; d2z ];
        % L'a _coup :
        d3y = -f^3*R*cos(f*t) ; d3x=0 ;
        d3z =  0;
        d3P = [ d3x ; d3y ; d3z ];
    case 2
        % La position 
        x = 0 ; y=0 ;
        z= A*cos(f*t) + B ; 
        P = [ x ; y ; z ];
        % La vitess
        dx = 0 ; dy=0 ;
        dz= -f*A*sin(f*t) ;
        dP = [ dx ; dy ; dz ];
        % L'acceleration :
        d2x = 0 ; d2y=0 ;
        d2z = -f^2*A*cos(f*t) ;
        d2P = [ d2x ; d2y ; d2z ];
        % L a_coup (jerk) :
        d3x = 0 ; d3y=0 ;
        d3z = f^3*A*sin(f*t) ;
        d3P = [ d3x ; d3y ; d3z ];
        
        %%
    case 3
        R=0.12;
        y = R*sin(f*t)  ; x=2*y;
        z= zpi  ;
        P = [ x ; y ; z ];
        % La vitess
        dy = f*R*cos(f*t)  ; dx=2*dy ;
        dz= 0 ;
        dP = [ dx ; dy ; dz ];
        % L'acceleration :
        d2y = -f^2*R*sin(f*t) ; d2x=2*d2y ;
        d2z =  0;
        d2P = [ d2x ; d2y ; d2z ];
        % L'a _coup :
        d3y = -f^3*R*cos(f*t) ; d3x=2*d3y ;
        d3z =  0;
        d3P = [ d3x ; d3y ; d3z ];
    case 4 % Cerecl XY
        x=R*cos(f*t) ; y=R*sin(f*t) ; z=zpi  ;
        dx=-f*R*sin(f*t) ; dy=f*R*cos(f*t)  ;  dz=0;
        d2x=-f^2*R*cos(f*t) ; d2y=-f^2*R*sin(f*t)  ;  d2z=0;
        P=[x ; y ; z];
        dP=[dx ; dy ; dz];
        d2P=[d2x ; d2y ; d2z];
        % L'a _coup :
        d3x=f^3*R*sin(f*t) ; d3y=-f^3*R*cos(f*t)  ;  d3z=0;
        d3P=[d3x ; d3y ; d3z];
        
    case 5 % ZY   
        x=0 ; y=R*sin(f*t) ; z=0.5*R*cos(f*t) + zpi  ;
        dx=0 ; dy=f*R*cos(f*t)  ;  dz=-f*0.5*R*sin(f*t);
        d2x=0 ; d2y=-f^2*R*sin(f*t)  ;  d2z=-f^2*0.5*R*cos(f*t);
        P=[x ; y ; z];
        dP=[dx ; dy ; dz];
        d2P=[d2x ; d2y ; d2z];
        d3x=0 ; d3y=-f^3*R*cos(f*t)  ;  d3z=f^3*0.5*R*sin(f*t);
        d3P=[d3x ; d3y ; d3z];
%     case 6 %Cercle ZX
%         y=0 ; x=R*sin(f*t) ; z=R*cos(f*t) +zpi;
%         dy=0 ; dx=f*R*cos(f*t)  ;  dz=-f*R*sin(f*t);
%         d2y=0 ; d2x=-f^2*R*sin(f*t)  ;  d2z=-f^2*R*cos(f*t);
%         d3y=0 ; d3x=-f^3*R*cos(f*t)  ;  d3z=f^3*R*sin(f*t);
%         P=[x ; y ; z];
%         dP=[dx ; dy ; dz];
%         d2P=[d2x ; d2y ; d2z];
%         d3P = [ d3x ; d3y ; d3z ];
%     case 7  % Les derivees sont a corriger
%         R=0.00*sin(f2*t) ; A=0.1270 ;
%         x=R*cos(f*t) ; y=R*sin(f*t) ;
%         z= A*sin(f2*t) -0.2 ;
%         dx=-f*R*sin(f*t) ; dy=f*R*cos(f*t)  ;  
%         dz= f2*A*cos(f2*t) ;
%         d2x=-f^2*R*cos(f*t) ; d2y=-f^2*R*sin(f*t)  ;
%         d2z = -f2^2*A*sin(f2*t) ;
%         P=[x ; y ; z];
%         dP=[dx ; dy ; dz];
%         d2P=[d2x ; d2y ; d2z];
%         % L'a _coup :
%         d3x=f^3*R*sin(f*t) ; d3y=-f^3*R*cos(f*t)  ;
%         d3z = -f2^3*A*cos(f2*t) ;
%         d3P=[d3x ; d3y ; d3z];
    case 8
        x=0 ; y=0 ; z=z0 ;
        P=[x ; y ; z];
        dP=[0 ; 0 ; 0];
        d2P=[0 ; 0 ; 0];
        d3P=[0 ; 0 ; 0];
        
    otherwise
        P=[0 ; 0 ; 0];
        dP=[0 ; 0 ; 0];
        d2P=[0 ; 0 ; 0];
        d3P = [ 0 ; 0 ; 0 ];
end

== matlab function Commande_3_Changement_de_base_et_diffeomorphisme_/RDelta_analityque/Moteurs/equations electriques ==
  data: I input; U input; dI output; dTheta input
function dI = fcn(I,U,dTheta)

% Les Constantes des moteurs ;

b1 = -1.1250e+03 ;
b2 = -99.4718 ;
b3 =833.3333 ;

dI = b2*dTheta + b1*I + b3*U ;
